simulink model "PubIfDecisionLSM_MDL"  (R2020b)
settings: configuration reference "DspaceConfig" (kept outside this file)
PostLoadFcn:
  | if any(exist('dsrtsu_mdlpostloadfcn', 'file') ~= 0), dsrtsu_mdlpostloadfcn('Execute', bdroot); end
InitFcn:
  | , if any(exist('rtifpga_mdlclblib', 'file') ~= 0), rtifpga_mdlclblib('Init', bdroot); end,
  | , if any(exist('dsmpb_private', 'file') ~= 0), dsmpb_private('dsmpb_mdlclblib', 'Init', bdroot); end,
values from neighbouring files (symbols this model uses):
  P_LSM_ALC_Enable = 0.0    [LSM_Parameter.sldd]
  P_LSM_AwayEdge_offset = 0.1    [LSM_Parameter.sldd]
  P_LSM_CentValidErr = 1.0    [LSM_Parameter.sldd]
  P_LSM_DOP_C0_EN_Limit = 0.8    [LSM_Parameter.sldd]
  P_LSM_DOP_C0_out_Limit = 2.0    [LSM_Parameter.sldd]
  P_LSM_DOP_C1_EN_Limit : value not decoded    [LSM_Parameter.sldd]
  P_LSM_DOP_C1_out_Limit : value not decoded    [LSM_Parameter.sldd]
  P_LSM_DOP_C1AndC2_Lim_X : value not decoded    [LSM_Parameter.sldd]
  P_LSM_DOP_C2_EN_Limit : value not decoded    [LSM_Parameter.sldd]
  P_LSM_DOP_C2_out_Limit : value not decoded    [LSM_Parameter.sldd]
  P_LSM_DOP_In_Pre2Dop_Dis = 1.0    [LSM_Parameter.sldd]
  P_LSM_DOP_Out_Pre2Dop_Dis = 2.0    [LSM_Parameter.sldd]
  P_LSM_DOP_PreDis_X : value not decoded    [LSM_Parameter.sldd]
  P_LSM_DOP_PreDis_Y : value not decoded    [LSM_Parameter.sldd]
  P_LSM_DOPEnableSW = 1.0    [LSM_Parameter.sldd]
  P_LSM_DOPValid_CheckTime = 0.06    [LSM_Parameter.sldd]
  P_LSM_DoubleLine_Curr2Cent_Dislimit = 0.5    [LSM_Parameter.sldd]
  P_LSM_DoubleLine_Dop2Cent_Dislimit = 0.5    [LSM_Parameter.sldd]
  P_LSM_DoubleLine_DOPOut_C1 : value not decoded    [LSM_Parameter.sldd]
  P_LSM_DoubleLine_Pre2Cent_Dislimit = 1.0    [LSM_Parameter.sldd]
  P_LSM_Error_Limit = 0.5    [LSM_Parameter.sldd]
  P_LSM_IFV2CenterAxis = 0.0    [LSM_Parameter.sldd]
  P_LSM_IFV2RearAxis = 0.0    [LSM_Parameter.sldd]
  P_LSM_Line2Edge_limit = 0.5    [LSM_Parameter.sldd]
  P_LSM_Line_Error = 0.1    [LSM_Parameter.sldd]
  P_LSM_LineSTD_Limit = 0.15    [LSM_Parameter.sldd]
  P_LSM_NOH_Switch = 0.0    [LSM_Parameter.sldd]
  P_LSM_OTL_C0_Factor = 1.0    [LSM_Parameter.sldd]
  P_LSM_OTL_C1_Factor = 0.5    [LSM_Parameter.sldd]
  P_LSM_OTL_C2_Factor = 0.5    [LSM_Parameter.sldd]
  P_LSM_Pre2OnlyLineDis = 5.0    [LSM_Parameter.sldd]
  P_LSM_Pre_t = 0.0    [LSM_Parameter.sldd]
  P_LSM_SingleLine_Cent2Edge_Dislimit = 100.0    [LSM_Parameter.sldd]
  P_LSM_SingleLine_Curr2Cent_Dislimit = 0.2    [LSM_Parameter.sldd]
  P_LSM_SingleLine_Dop2Cent_Dislimit = 0.2    [LSM_Parameter.sldd]
  P_LSM_SingleLine_DOPOut_C1 : value not decoded    [LSM_Parameter.sldd]
  P_LSM_SingleLine_Pre2Cent_Dislimit = 0.5    [LSM_Parameter.sldd]
  P_LSM_TJALimitSpd = 60.0    [LSM_Parameter.sldd]
undefined symbols (not defined in the file or in its folder): P_lCS_IFV2CenterAxis, P_LCS_IFV2RearAxis, P_LSM_EntryEdge_offset, P_LSM_EntryLnChngEnSwitch, P_LSM_EntryVanishDis, P_LSM_LinetLostTime, P_LSM_LineWijCal_C12, P_LSM_LineWijCal_C13, P_LSM_MapValid_ErrorSwitch, P_LSM_PosLineLcFac, P_LSM_SpdLim_Stub_Spd, P_LSM_SpdLim_StubLength, P_LSM_SpdTurnAlarm
libraries: simulink x324, TrueDurationTime x11
(part 9 of 25)

== system PubIfDecisionLSM_MDL/Subsystem1/TargetLineCalc_20ms/TargetLineCalc/Subsystem5 ==
  kap : Inport
  vRef : Inport  Port=2
  preDis : Inport  Port=3
  RoadWidth1 : Inport  Port=4
  <CentLineValid> : Inport  Port=5
  <CentLineC3> : Inport  Port=6
  <CentLineC2> : Inport  Port=7
  <CentLineC1> : Inport  Port=8
  <CentLineC0> : Inport  Port=9
  Conf : Inport  Port=10
  <A3> : Inport  Port=11
  <A2> : Inport  Port=12
  <A1> : Inport  Port=13
  <A0> : Inport  Port=14
  <LineReliable> : Inport  Port=15
  <Range> : Inport  Port=16
  CosOfPsi : Inport  Port=17
  SinOfPsi : Inport  Port=18
  dDeltaX : Inport  Port=19
  dDeltaY : Inport  Port=20
  HWASts : Inport  Port=21
  1-D Lookup Table3 : Lookup_n-D  NumberOfTableDimensions=1  BreakpointsForDimension1=[0 0.0001 0.0005 0.001 0.005 0.01 0.05]  Table=[0 0.1 0.3 0.6 0.8 0.8 0.8]  InternalRulePriority=Speed  RndMeth=Simplest  InputSameDT=on
  1-D Lookup Table4 : Lookup_n-D  NumberOfTableDimensions=1  BreakpointsForDimension1=[0 0.0001 0.0005 0.001 0.005 0.01 0.05]  Table=[0 0.1 0.3 0.6 0.8 0.8 0.8]  InternalRulePriority=Speed  RndMeth=Simplest  InputSameDT=on
  1-D Lookup Table5 : Lookup_n-D  NumberOfTableDimensions=1  BreakpointsForDimension1=[0 0.1 0.3 0.5 0.7 0.9 1]  Table=[0 0.1 0.2 0.4 0.7 1 1]  InternalRulePriority=Speed  RndMeth=Simplest  InputSameDT=on
  1-D Lookup Table6 : Lookup_n-D  NumberOfTableDimensions=1  BreakpointsForDimension1=[0 0.1 0.3 0.5 0.7 0.9 1]  Table=[0 0.1 0.2 0.4 0.7 1 1]  InternalRulePriority=Speed  RndMeth=Simplest  InputSameDT=on
  2-D Lookup Table : Lookup_n-D  BreakpointsForDimension1=[20,50,100,120]  BreakpointsForDimension2=[0,0.2,0.4,0.6,0.8,1,1.2,1.4,1.6,1.8,2,2.5,3]  Table=reshape([1,1,1,1,1,1,1,1,1,1,1,1,1,1,1,0.8,1,0.9,0.5,0.4,1,0.8,0.3,0.2,1,0.7,0.1,0.1,1,0.6,0,0,0.8,0.5,0,0,0.7,0.3,0,0,0.6,0,0,0,0.3,0,0,0,0,0,0,0],4,13)  InternalRulePriority=Speed  RndMeth=Simplest  InputSameDT=on
      settings: InputPortMap=u0,u1
  2-D Lookup Table1 : Lookup_n-D  BreakpointsForDimension1=[20,50,100,120]  BreakpointsForDimension2=[0,0.2,0.4,0.6,0.8,1,1.2,1.4,1.6,1.8,2,2.5,3]  Table=reshape([1,1,1,1,1,1,1,1,1,1,1,1,1,1,1,0.8,1,0.9,0.5,0.4,1,0.8,0.3,0.2,1,0.7,0.1,0.1,1,0.6,0,0,0.8,0.5,0,0,0.7,0.3,0,0,0.6,0,0,0,0.3,0,0,0,0,0,0,0],4,13)  InternalRulePriority=Speed  RndMeth=Simplest  InputSameDT=on
      settings: InputPortMap=u0,u1
  2-D Lookup Table2 : Lookup_n-D  Commented=on  BreakpointsForDimension1=[20,50,100]  BreakpointsForDimension2=[0,0.2,0.4,0.6,0.8,1,1.2,1.4,1.6,1.8,2,2.5,3]  Table=reshape([1,1,1,1,1,1,1,1,0.9,1,1,0.5,1,0.9,0.3,1,0.8,0.2,1,0.7,0.1,1,0.6,0,0.8,0.5,0,0.7,0.3,0,0.6,0.1,0,0.3,0,0,0,0,0],3,13)  InternalRulePriority=Speed  RndMeth=Simplest  InputSameDT=on
      settings: InputPortMap=u0,u1
  2-D Lookup Table3 : Lookup_n-D  BreakpointsForDimension1=[10,50,80,120]  BreakpointsForDimension2=[0,5,10,20,40,50,60,80,100]  Table=reshape([0,0,0,0,0,0,0,0,0.4,0.2,0,0,0.6,0.4,0.2,0,1,0.6,0.5,0.3,1,0.8,0.7,0.5,1,1,0.9,0.8,1,1,1,1,1,1,1,1],4,9)  InternalRulePriority=Speed  RndMeth=Simplest  InputSameDT=on
      settings: InputPortMap=u0,u1
  2-D Lookup Table4 : Lookup_n-D  BreakpointsForDimension1=[10,50,80,120]  BreakpointsForDimension2=[0,5,10,20,40,50,60,80,100]  Table=reshape([0,0,0,0,0,0,0,0,0.4,0.2,0,0,0.6,0.4,0.2,0,1,0.6,0.5,0.3,1,0.8,0.7,0.5,1,1,0.9,0.8,1,1,1,1,1,1,1,1],4,9)  InternalRulePriority=Speed  RndMeth=Simplest  InputSameDT=on
      settings: InputPortMap=u0,u1
  <A2>1 : InportShadow  Port=12
  Abs2 : Abs
  Abs3 : Abs
  Add : Sum  Inputs=+++
  Add1 : Sum  Inputs=+++
  Constant10 : Constant  Value=[0,0,0.2,0.5,0.8,1,1,1,1,0.3,0,0]
  Constant11 : Constant  Value=[-1.2,-0.2,0,0.5,1,1.3,1.5,2.1,2.3,3.5,4,5]
  Constant12 : Constant  Value=3.75
  Constant13 : Constant  Value=[0,0,0.2,0.5,0.8,1,1,1,1,0.3,0,0]
  Constant14 : Constant  Value=[-1.2,-0.2,0,0.5,1,1.3,1.5,2.1,2.3,3.5,4,5]
  Constant15 : Constant  Value=3.75
  Constant16 : Constant  Value=1.3  OutDataTypeStr=single
  Constant21 : Constant  Value=1.3  OutDataTypeStr=single
  Constant7 : Constant  Value=P_LSM_LineWijCal_C12
  Constant9 : Constant  Value=P_LSM_LineWijCal_C13
  Gain1 : Gain  Gain=3.6
  Gain2 : Gain  Gain=1.03
  Gain3 : Gain  Gain=3.6
  Gain4 : Gain  Gain=1.03
  If : If
  If Action Subsystem : Subsystem  TreatAsAtomicUnit=on
  If Action Subsystem1 : Subsystem  TreatAsAtomicUnit=on
  If Action Subsystem2 : Subsystem  TreatAsAtomicUnit=on
  If Action Subsystem3 : Subsystem  TreatAsAtomicUnit=on
  If Action Subsystem4 : Subsystem  TreatAsAtomicUnit=on
  If Action Subsystem5 : Subsystem  TreatAsAtomicUnit=on
  If1 : If
  If2 : If
  Lookup Table Dynamic : simulink/Lookup Tables/Lookup Table Dynamic  LookUpMeth=Interpolation-Use End Values  OutDataType=fixdt('single')  OutScaling=[]  OutputDataTypeScalingMode=Specify via dialog  OutDataTypeStr=single  DoSatur=off
  Lookup Table Dynamic1 : simulink/Lookup Tables/Lookup Table Dynamic  LookUpMeth=Interpolation-Use End Values  OutDataType=fixdt('single')  OutScaling=[]  OutputDataTypeScalingMode=Specify via dialog  OutDataTypeStr=single  DoSatur=off
  MATLAB Function2 : MATLAB Function  TreatAsAtomicUnit=on
  MATLAB Function3 : MATLAB Function  TreatAsAtomicUnit=on
  MATLAB Function6 : MATLAB Function  TreatAsAtomicUnit=on
  MATLAB Function7 : MATLAB Function  TreatAsAtomicUnit=on
  MATLAB Function8 : MATLAB Function  TreatAsAtomicUnit=on
  Merge{,1..3} (4 alike) : Merge
  Product{,1..7} (8 alike) : Product
  Product8 : Product  Inputs=**/
  Product9 : Product  Inputs=**/
  RoadWidth1_1 : InportShadow  Port=4
  Saturation : Saturate  UpperLimit=single(5)  LowerLimit=single(2.4)
  Saturation1 : Saturate  UpperLimit=single(5)  LowerLimit=single(2.4)
  Selector2 : Selector  InputPortWidth=4  IndexOptions=Index vector (dialog)  Indices=2  OutputSizes=1
  Selector3 : Selector  InputPortWidth=4  IndexOptions=Index vector (dialog)  Indices=3  OutputSizes=1
  Selector4 : Selector  InputPortWidth=4  IndexOptions=Index vector (dialog)  Indices=2  OutputSizes=1
  Selector5 : Selector  InputPortWidth=4  IndexOptions=Index vector (dialog)  Indices=3  OutputSizes=1
  Selector6 : Selector  InputPortWidth=4  IndexOptions=Index vector (dialog)  Indices=2  OutputSizes=1
  Selector7 : Selector  InputPortWidth=4  IndexOptions=Index vector (dialog)  Indices=3  OutputSizes=1
  Sum : Sum  Inputs=|++
  Sum1 : Sum  Inputs=|++
  Unit Delay : UnitDelay  SampleTime=-1  HasFrameUpgradeWarning=on
  Unit Delay1 : UnitDelay  SampleTime=-1  HasFrameUpgradeWarning=on
  vRef_1 : InportShadow  Port=2
  LH1Wij : Outport
  LH2Wij : Outport  Port=2
  wires:
  Saturation1/1 -> Product9/2
  RoadWidth1/1 -> Saturation/1
  [LH22] -> Product2/1
  Lookup Table Dynamic1/1 -> Product4/1
  Gain1/1 -> Gain2/1
  [LH21] -> Product1/1
  <CentLineC0>/1 -> MATLAB Function6/7(CentLineC0K1)
  Gain2/1 -> Sum1/1
  Product/1 -> [LH21]
  <Range>/1 -> Selector3/1, Selector2/1
  Saturation/1 -> Product8/2
  vRef_1/1 -> Gain1/1
  MATLAB Function6/1(d_cur2) -> Lookup Table Dynamic/1
  2-D Lookup Table1/1 -> Product4/2
  <LineReliable>/1 -> MATLAB Function8/1(VisLineReliable)
  Sum1/1 -> 2-D Lookup Table4/1, 2-D Lookup Table3/1
  Product5/1 -> Add1/1
  1-D Lookup Table5/1 -> [LH23]
  Product7/1 -> Add1/3
  [LH33] -> Product7/1
  dDeltaX/1 -> MATLAB Function6/16(dDeltaX)
  MATLAB Function8/2(dy3_Rel) -> 1-D Lookup Table6/1
  Constant16/1 -> Sum/2
  Constant13/1 -> Lookup Table Dynamic1/3
  Constant21/1 -> Sum1/2
  MATLAB Function3/1(Fac1) -> [Fac1]
  2-D Lookup Table3/1 -> [LH22]
  Sum/1 -> 2-D Lookup Table1/1, 2-D Lookup Table/1
  Constant12/1 -> Product8/3
  [Fac3] -> Product7/2
  [Fac1] -> Product5/2
  [Fac2] -> Product6/2
  <CentLineC2>/1 -> MATLAB Function6/5(CentLineC2K1)
  [LH23] -> Product3/1
  SinOfPsi/1 -> MATLAB Function6/15(SinOfPsi)
  Product8/1 -> Lookup Table Dynamic/2
  1-D Lookup Table6/1 -> [LH33]
  Product2/1 -> Add/2
  [Fac1] -> Product1/2
  Product1/1 -> Add/1
  2-D Lookup Table/1 -> Product/2
  <CentLineC1>/1 -> MATLAB Function6/6(CentLineC1K1)
  Selector2/1 -> MATLAB Function7/1(L2_R)
  Product9/1 -> Lookup Table Dynamic1/2
  Gain3/1 -> Gain4/1
  <A0>/1 -> MATLAB Function6/11(VisLineA0)
  Constant11/1 -> Product8/1
  Product6/1 -> Add1/2
  Gain4/1 -> Sum/1
  MATLAB Function6/3(d_cur3) -> Lookup Table Dynamic1/1
  MATLAB Function6/2(delta_d2) -> 2-D Lookup Table/2
  RoadWidth1_1/1 -> Saturation1/1
  Constant14/1 -> Product9/1
  Lookup Table Dynamic/1 -> Product/1
  Constant10/1 -> Lookup Table Dynamic/3
  <CentLineC3>/1 -> MATLAB Function6/4(CentLineC3K1)
  [LH32] -> Product6/1
  MATLAB Function6/4(delta_d3) -> 2-D Lookup Table1/2
  [Fac2] -> Product2/2
  Constant9/1 -> MATLAB Function3/2(C13)
  [LH31] -> Product5/1
  [Fac3] -> Product3/2
  Constant7/1 -> MATLAB Function3/1(C12)
  Constant15/1 -> Product9/3
  MATLAB Function7/1(dy2_Ran) -> 2-D Lookup Table3/2
  MATLAB Function8/1(dy2_Rel) -> 1-D Lookup Table5/1
  preDis/1 -> MATLAB Function6/2(preDis)
  MATLAB Function3/2(Fac2) -> [Fac2]
  Product4/1 -> [LH31]
  vRef/1 -> Gain3/1
  MATLAB Function3/3(Fac3) -> [Fac3]
  kap/1 -> MATLAB Function6/1(kap)
  2-D Lookup Table4/1 -> [LH32]
  MATLAB Function7/2(dy3_Ran) -> 2-D Lookup Table4/2
  Product3/1 -> Add/3
  <A2>/1 -> MATLAB Function6/9(VisLineA2)
  Selector3/1 -> MATLAB Function7/2(L3_R)
  CosOfPsi/1 -> MATLAB Function6/14(CosOfPsi)
  <A1>/1 -> MATLAB Function6/10(VisLineA1)
  <A3>/1 -> MATLAB Function6/8(VisLineA3)
  dDeltaY/1 -> MATLAB Function6/17(dDeltaY)
  Conf/1 -> Selector5/1, Selector4/1
  Selector5/1 -> If1/1
  Selector4/1 -> If/1
  Add/1 -> If Action Subsystem/1(In1)
  If/2 -> If Action Subsystem2/Action
  Merge/1 -> LH1Wij/1
  If Action Subsystem/1(LH1Wij) -> Merge/1
  If Action Subsystem2/1(LH1Wij) -> Merge/2
  If Action Subsystem3/1(LH1Wij) -> Merge1/2
  If Action Subsystem1/1(LH1Wij) -> Merge1/1
  Merge1/1 -> LH2Wij/1
  Add1/1 -> If Action Subsystem1/1(In1)
  If1/2 -> If Action Subsystem3/Action
  If/1 -> If Action Subsystem/Action
  If1/1 -> If Action Subsystem1/Action
  <CentLineValid>/1 -> MATLAB Function6/3(CentLineValidK1)
  If Action Subsystem5/2(Out2) -> Merge3/1
  1-D Lookup Table4/1 -> If Action Subsystem4/1(In1)
  If2/2 -> If Action Subsystem4/Action
  If Action Subsystem4/2(Out2) -> Merge3/2
  Merge2/1 -> MATLAB Function6/12(n1)
  If Action Subsystem4/1(Out1) -> Merge2/2
  Abs2/1 -> 1-D Lookup Table4/1
  <A2>1/1 -> Selector7/1, Selector6/1
  Abs3/1 -> 1-D Lookup Table3/1
  1-D Lookup Table3/1 -> If Action Subsystem4/2(In2)
  If2/1 -> If Action Subsystem5/Action
  If Action Subsystem5/1(Out1) -> Merge2/1
  Merge3/1 -> MATLAB Function6/13(n2)
  Selector6/1 -> Abs2/1
  Selector7/1 -> Abs3/1
  Unit Delay1/1 -> MATLAB Function2/2(HWAStsK1)
  HWASts/1 -> MATLAB Function6/18(HWASts), MATLAB Function2/1(HWASts), Unit Delay1/1
  MATLAB Function2/1(Changelane) -> If2/1
  MATLAB Function2/2(Lock_counter) -> Unit Delay/1
  Unit Delay/1 -> MATLAB Function2/3(Lock_counterK1)

== system PubIfDecisionLSM_MDL/Subsystem1/TargetLineCalc_20ms/TargetLineCalc/TypeConf ==
  LeftType : Inport
  LeftDLMType : Inport  Port=2
  LeftDECELType : Inport  Port=3
  RightType : Inport  Port=4
  RightDLMType : Inport  Port=5
  RightDECELType : Inport  Port=6
  Line_update : Inport  Port=7
  LeftColor : Inport  Port=8
  LLeftType : Inport  Port=9
  MATLAB Function : MATLAB Function  TreatAsAtomicUnit=on
  RoadWidthCalc1 : MATLAB Function  TreatAsAtomicUnit=on
  Unit Delay{,1..7,36..37} (10 alike) : UnitDelay  SampleTime=-1  HasFrameUpgradeWarning=on
  Out1 : Outport
  Out2 : Outport  Port=2
  wires:
  MATLAB Function/7(LeftColor) -> Unit Delay6/1
  MATLAB Function/4(RightType) -> RoadWidthCalc1/4(RightType), Unit Delay2/1
  LeftColor/1 -> MATLAB Function/8(LeftColor_en)
  Unit Delay3/1 -> MATLAB Function/14(RightDLMTypeK1)
  Unit Delay7/1 -> MATLAB Function/17(LLeftType_enK1)
  Unit Delay6/1 -> MATLAB Function/16(LeftColor_enK1)
  LeftDLMType/1 -> MATLAB Function/3(LeftDLMType_en)
  Unit Delay5/1 -> MATLAB Function/12(LeftDECELTypeK1)
  Unit Delay4/1 -> MATLAB Function/15(RightDECELTypeK1)
  Unit Delay2/1 -> MATLAB Function/13(RightTypeK1)
  MATLAB Function/8(LLeftType) -> Unit Delay7/1
  Unit Delay1/1 -> MATLAB Function/11(LeftDLMTypeK1)
  LeftDECELType/1 -> MATLAB Function/4(LeftDECELType_en)
  RightDECELType/1 -> MATLAB Function/7(RightDECELType_en)
  MATLAB Function/6(RightDECELType) -> RoadWidthCalc1/6(RightDECELType), Unit Delay4/1
  MATLAB Function/5(RightDLMType) -> RoadWidthCalc1/5(RightDLMType), Unit Delay3/1
  MATLAB Function/1(LeftType) -> Unit Delay/1, RoadWidthCalc1/1(LeftType)
  LLeftType/1 -> MATLAB Function/9(LLeftType_en)
  RoadWidthCalc1/1(LeftEn) -> Out1/1
  Unit Delay36/1 -> RoadWidthCalc1/8(Cnt2K1)
  Unit Delay37/1 -> RoadWidthCalc1/7(Cnt1K1)
  MATLAB Function/2(LeftDLMType) -> Unit Delay1/1, RoadWidthCalc1/2(LeftDLMType)
  MATLAB Function/3(LeftDECELType) -> Unit Delay5/1, RoadWidthCalc1/3(LeftDECELType)
  RoadWidthCalc1/4(Cnt2) -> Unit Delay36/1
  RightType/1 -> MATLAB Function/5(RightType_en)
  RoadWidthCalc1/3(Cnt1) -> Unit Delay37/1
  LeftType/1 -> MATLAB Function/2(LeftType_en)
  Unit Delay/1 -> MATLAB Function/10(LeftTypeK1)
  RightDLMType/1 -> MATLAB Function/6(RightDLMType_en)
  Line_update/1 -> MATLAB Function/1(update)
  RoadWidthCalc1/2(RightEn) -> Out2/1

== system PubIfDecisionLSM_MDL/Subsystem1/TargetLineCalc_20ms/TargetLineCalc/TypeConf1 ==
  LeftType : Inport
  RightType : Inport  Port=2
  RoadWidthCalc1 : MATLAB Function  TreatAsAtomicUnit=on
  Unit Delay36 : UnitDelay  SampleTime=-1  HasFrameUpgradeWarning=on
  Unit Delay37 : UnitDelay  SampleTime=-1  HasFrameUpgradeWarning=on
  LeftEn : Outport
  RightEn : Outport  Port=2
  wires:
  RightType/1 -> RoadWidthCalc1/2(RightType)
  Unit Delay36/1 -> RoadWidthCalc1/4(Cnt2K1)
  RoadWidthCalc1/2(RightEn) -> RightEn/1
  LeftType/1 -> RoadWidthCalc1/1(LeftType)
  RoadWidthCalc1/4(Cnt2) -> Unit Delay36/1
  RoadWidthCalc1/3(Cnt1) -> Unit Delay37/1
  Unit Delay37/1 -> RoadWidthCalc1/3(Cnt1K1)
  RoadWidthCalc1/1(LeftEn) -> LeftEn/1

== system PubIfDecisionLSM_MDL/Subsystem1/TargetLineCalc_20ms2/TargetLineCalc/CenLineCal1 ==
  LCKSts : Inport
  kap : Inport  Port=2
  preDis : Inport  Port=3
  VisLine : Inport  Port=4
  VisEdge : Inport  Port=5
  RoadWidth : Inport  Port=6
  LeftLane_change : Inport  Port=7
  RightLane_change : Inport  Port=8
  Bus Creator2 : BusCreator  Inputs=7
  Bus Selector1 : BusSelector  OutputSignals=EdgeConf,EdgeA3,EdgeA2,EdgeA1,EdgeA0
  Bus Selector5 : BusSelector  OutputSignals=LineConf,LineReliable,A3,A2,A1,A0,Range
  Constant : Constant  Value=P_LSM_Line_Error
  Constant1 : Constant  Value=P_LSM_Line2Edge_limit
  Constant2 : Constant  Value=P_LSM_AwayEdge_offset
  Constant3 : Constant  Value=P_LSM_Pre2OnlyLineDis
  Constant4 : Constant  Value=P_LSM_CentValidErr
  Constant5 : Constant  Value=0  OutDataTypeStr=boolean
  Constant6 : Constant  Value=0  OutDataTypeStr=uint8
  Switch : Switch  Criteria=u2 > Threshold
  Switch1 : Switch  Criteria=u2 > Threshold
  Terminator : Terminator
  Unit Delay : UnitDelay  SampleTime=-1  HasFrameUpgradeWarning=on
  Unit Delay1 : UnitDelay  SampleTime=-1  HasFrameUpgradeWarning=on
  centerLineFilter : MATLAB Function  TreatAsAtomicUnit=on
  CenLine : Outport
  Double_Line_Lost : Outport  Port=2
  Line_State : Outport  Port=3
  wires:
  Switch1/1 -> Line_State/1
  Constant6/1 -> Switch1/3
  Switch/1 -> Bus Creator2/1  "CentLineConf"
  Constant5/1 -> Switch/3
  Constant4/1 -> Switch/2, Switch1/2
  Constant3/1 -> centerLineFilter/22(Pre2OnlyLineDis)
  RightLane_change/1 -> centerLineFilter/2(RightLane_change)
  LeftLane_change/1 -> centerLineFilter/1(LeftLane_change)
  centerLineFilter/7(CenLineReliable) -> Bus Creator2/7
  Bus Selector5/2 -> centerLineFilter/10(LineReliable)  "<LineReliable>"
  Constant2/1 -> centerLineFilter/5(Away_offset)
  Constant1/1 -> centerLineFilter/4(Edge_error)
  centerLineFilter/10(Offset) -> Terminator/1  "LSM_Edge_Offset"
  Unit Delay1/1 -> centerLineFilter/24(R_CounterK1)
  Unit Delay/1 -> centerLineFilter/23(L_CounterK1)
  centerLineFilter/12(R_Counter) -> Unit Delay1/1
  centerLineFilter/11(L_Counter) -> Unit Delay/1
  Constant/1 -> centerLineFilter/3(Line_error)
  centerLineFilter/9(Double_Line_Lost) -> Double_Line_Lost/1
  LCKSts/1 -> centerLineFilter/6(LCKSts)
  kap/1 -> centerLineFilter/7(kap)
  RoadWidth/1 -> centerLineFilter/21(RoadWidth)
  Bus Selector1/5 -> centerLineFilter/20(VisEdgeA0)  "<EdgeA0>"
  Bus Selector1/4 -> centerLineFilter/19(VisEdgeA1)  "<EdgeA1>"
  Bus Selector1/3 -> centerLineFilter/18(VisEdgeA2)  "<EdgeA2>"
  Bus Selector1/2 -> centerLineFilter/17(VisEdgeA3)  "<EdgeA3>"
  Bus Selector1/1 -> centerLineFilter/16(VisEdgeConf)  "<EdgeConf>"
  Bus Selector5/7 -> centerLineFilter/15(VisLineR)  "<Range>"
  Bus Selector5/6 -> centerLineFilter/14(VisLineA0)  "<A0>"
  Bus Selector5/1 -> centerLineFilter/9(VisLineConf)  "<LineConf>"
  Bus Selector5/5 -> centerLineFilter/13(VisLineA1)  "<A1>"
  Bus Selector5/3 -> centerLineFilter/11(VisLineA3)  "<A3>"
  Bus Selector5/4 -> centerLineFilter/12(VisLineA2)  "<A2>"
  preDis/1 -> centerLineFilter/8(preDis)
  centerLineFilter/8(Line_State) -> Switch1/1  "LSM_Line_state"
  VisEdge/1 -> Bus Selector1/1
  Bus Creator2/1 -> CenLine/1
  centerLineFilter/5(CentLineC0) -> Bus Creator2/5
  centerLineFilter/3(CentLineC2) -> Bus Creator2/3
  centerLineFilter/1(CentLineConf) -> Switch/1
  centerLineFilter/6(CentLineRange) -> Bus Creator2/6
  VisLine/1 -> Bus Selector5/1
  centerLineFilter/2(CentLineC3) -> Bus Creator2/2
  centerLineFilter/4(CentLineC1) -> Bus Creator2/4

== system PubIfDecisionLSM_MDL/Subsystem1/TargetLineCalc_20ms2/TargetLineCalc/DetectChange ==
  OTLCount : Inport
  Relational Operator : RelationalOperator  Operator=~=  OutDataTypeStr=boolean  RndMeth=Simplest
  Unit Delay49 : UnitDelay  InitialCondition=uint8(0)  SampleTime=-1  HasFrameUpgradeWarning=on
  Out1 : Outport
  wires:
  Relational Operator/1 -> Out1/1
  OTLCount/1 -> Unit Delay49/1, Relational Operator/2
  Unit Delay49/1 -> Relational Operator/1

== system PubIfDecisionLSM_MDL/Subsystem1/TargetLineCalc_20ms2/TargetLineCalc/DetectChange1 ==
  In1 : Inport
  Constant : Constant  Value=0  OutDataTypeStr=uint8
  Relational Operator1 : RelationalOperator  Operator=~=  OutDataTypeStr=boolean  RndMeth=Simplest
  Switch : Switch  Criteria=u2 > Threshold
  Unit Delay68 : UnitDelay  SampleTime=-1  HasFrameUpgradeWarning=on
  Out1 : Outport
  wires:
  Constant/1 -> Switch/3
  Switch/1 -> Out1/1
  Relational Operator1/1 -> Switch/2
  In1/1 -> Relational Operator1/1, Switch/1, Unit Delay68/1
  Unit Delay68/1 -> Relational Operator1/2

== system PubIfDecisionLSM_MDL/Subsystem1/TargetLineCalc_20ms2/TargetLineCalc/DetectIncrease ==
  In : Inport
  Relational Operator : RelationalOperator  Operator=>  OutDataTypeStr=boolean  RndMeth=Simplest
  Unit Delay67 : UnitDelay  SampleTime=-1  HasFrameUpgradeWarning=on
  Out : Outport
  wires:
  Relational Operator/1 -> Out/1
  In/1 -> Relational Operator/1, Unit Delay67/1
  Unit Delay67/1 -> Relational Operator/2

== system PubIfDecisionLSM_MDL/Subsystem1/TargetLineCalc_20ms2/TargetLineCalc/DetectIncrease1 ==
  In : Inport
  Relational Operator : RelationalOperator  Operator=>  OutDataTypeStr=boolean  RndMeth=Simplest
  Unit Delay67 : UnitDelay  SampleTime=-1  HasFrameUpgradeWarning=on
  out : Outport
  wires:
  Unit Delay67/1 -> Relational Operator/2
  In/1 -> Unit Delay67/1, Relational Operator/1
  Relational Operator/1 -> out/1

== system PubIfDecisionLSM_MDL/Subsystem1/TargetLineCalc_20ms2/TargetLineCalc/Subsystem ==
  Spd : Inport
  Compare To Constant22 : simulink/Logic and Bit Operations/Compare To Constant  relop=<  const=1  OutDataTypeStr=boolean
  Constant21 : Constant  Value=0xff
  Switch10 : Switch
  Out1 : Outport
  wires:
  Switch10/1 -> Out1/1
  Constant21/1 -> Switch10/1
  Spd/1 -> Switch10/3, Compare To Constant22/1
  Compare To Constant22/1 -> Switch10/2

== system PubIfDecisionLSM_MDL/Subsystem1/TargetLineCalc_20ms2/TargetLineCalc/Subsystem1 ==
  Dis : Inport
  Compare To Constant1 : simulink/Logic and Bit Operations/Compare To Constant  relop=>  const=2000  OutDataTypeStr=boolean
  Compare To Constant22 : simulink/Logic and Bit Operations/Compare To Constant  relop=<  const=1  OutDataTypeStr=boolean
  Constant21 : Constant  Value=0xffff
  OR : Logic  Operator=OR  AllPortsSameDT=off  OutDataTypeStr=boolean
  Switch10 : Switch
  Out1 : Outport
  wires:
  OR/1 -> Switch10/2
  Compare To Constant1/1 -> OR/2
  Compare To Constant22/1 -> OR/1
  Dis/1 -> Compare To Constant22/1, Compare To Constant1/1, Switch10/3
  Constant21/1 -> Switch10/1
  Switch10/1 -> Out1/1

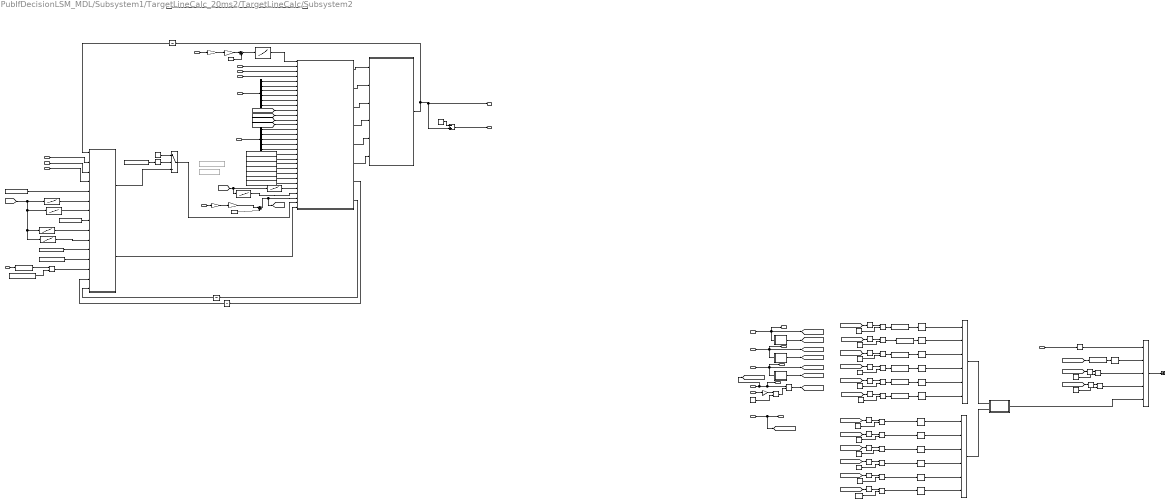
== system PubIfDecisionLSM_MDL/Subsystem1/TargetLineCalc_20ms2/TargetLineCalc/Subsystem2 ==
  LCKSts : Inport
  Line_State : Inport  Port=2
  vRef : Inport  Port=3
  DOP_Valid : Inport  Port=4
  DOP_C3 : Inport  Port=5
  DOP_C2 : Inport  Port=6
  DOP_C1 : Inport  Port=7
  DOP_C0 : Inport  Port=8
  DOP_Range : Inport  Port=9
  CentLine : Inport  Port=10
  EdgeLine : Inport  Port=11
  kap : Inport  Port=12
  Abs{,1,3..14} (14 alike) : Abs
  Bus Selector1 : BusSelector  OutputSignals=EdgeConf,EdgeA3,EdgeA2,EdgeA1,EdgeA0
  Bus Selector6 : BusSelector  OutputSignals=CentLineConf,CentLineC3,CentLineC2,CentLineC1,CentLineC0,CentLineRange
  C0max : Constant  Value=1.5  OutDataTypeStr=single
  C0th : Constant  Value=0.9  OutDataTypeStr=single
  C0th1 : Constant  Value=0.6  OutDataTypeStr=single
  C1max:30° : Constant  Value=0.58  OutDataTypeStr=single
  C1th:10° : Constant  Value=0.176  OutDataTypeStr=single
  C1th:10°1 : Constant  Value=0.08  OutDataTypeStr=single
  C2th : Constant  Value=0.008  OutDataTypeStr=single
  C2th1 : Constant  Value=0.006  OutDataTypeStr=single
  Chart : Stateflow chart  TreatAsAtomicUnit=on
      settings: PortSchema="{\"entries\":[{\"content\":{\"sides\":[{\"content\":{\"connectorIds\":[\"In2\",\"In1\"]},\"type\":\"ConnectorPlacement.EquallySpacedRectSide\",\"uuid\":\"e53ab263-18d4-4398-8fad-2a536e7c737c\"},{\"content\":{\"connectorIds\":[\"Out1\"],\"side\":\"RIGHT\"},\"type\":\"ConnectorPlacement.EquallySpacedRectSide\",\"uuid\":\"b2acecce-e73e-419a-a9e7-11eb92620f5a\"},{\"content\":{\"connectorIds\":[],\"side\":\"TOP\"},\"type\":\"ConnectorPlacement.EquallySpacedRectSide\",\"uuid\":\"8139e609-291b-42df-ade2-518731258890\"},{\"content\":{\"connectorIds\":[],\"side\":\"HIDDEN\"},\"type\":\"ConnectorPlacement.EquallySpacedRectSide\",\"uuid\":\"25f8d80a-ba71-4848-a7f0-1c840b95c0bf\"}]},\"type\":\"ConnectorPlacement.EquallySpacedConnector\",\"uuid\":\"d97a9ee1-ef81-44f0-bee3-63dee7baeb52\"}],\"packageUris\":[\"http://schema.mathworks.com/mf0/Connector/R2020b\"],\"version\":\"1.0\"}"
  Compare To Constant{,1,9..14} (8 alike) : simulink/Logic and Bit Operations/Compare To Constant  relop===  const=1  OutDataTypeStr=boolean
  Compare To Constant{2,4,6,8} (4 alike) : simulink/Logic and Bit Operations/Compare To Constant  relop=>  const=0.1  OutDataTypeStr=boolean
  Compare To Constant3 : simulink/Logic and Bit Operations/Compare To Constant  relop=>  const=0.06  OutDataTypeStr=boolean
  Compare To Constant5 : simulink/Logic and Bit Operations/Compare To Constant  relop=>  const=0.06  OutDataTypeStr=boolean
  Compare To Constant7 : simulink/Logic and Bit Operations/Compare To Constant  relop=>  const=0.06  OutDataTypeStr=boolean
  Constant : Constant  Value=P_LSM_DOPEnableSW
  Constant1 : Constant  OutDataTypeStr=boolean
  Constant10 : Constant  Commented=on  Value=P_LSM_Error_Limit
  Constant11 : Constant  Value=1.3  OutDataTypeStr=single
  Constant12 : Constant  Commented=on  Value=P_LSM_TJALimitSpd
  Constant13 : Constant  Value=P_LSM_DoubleLine_Dop2Cent_Dislimit
  Constant14 : Constant  Value=P_LSM_DOP_In_Pre2Dop_Dis
  Constant15 : Constant  OutDataTypeStr=uint8
  Constant16 : Constant  Value=P_LSM_SingleLine_Cent2Edge_Dislimit
  Constant17 : Constant  Value=P_LSM_SingleLine_Pre2Cent_Dislimit
  Constant18 : Constant  Value=P_LSM_SingleLine_Curr2Cent_Dislimit
  Constant19 : Constant  Value=P_LSM_DoubleLine_Pre2Cent_Dislimit
  Constant2 : Constant  Value=25  OutDataTypeStr=single
  Constant20 : Constant  Value=P_LSM_DoubleLine_Curr2Cent_Dislimit
  Constant21 : Constant  Value=P_LSM_SingleLine_Dop2Cent_Dislimit
  Constant22 : Constant  Value=P_LSM_DOP_Out_Pre2Dop_Dis
  Constant23 : Constant  Value=P_LSM_DOPValid_CheckTime
  Constant3 : Constant  Value=P_LSM_DOP_C0_EN_Limit
  Constant6 : Constant  Value=P_LSM_DOP_C0_out_Limit
  Constant9 : Constant  Value=1.3  OutDataTypeStr=single
  DOP_C4 : InportShadow  Port=8
  DOP_C5 : InportShadow  Port=7
  DOP_C6 : InportShadow  Port=6
  DOP_Valid1 : InportShadow  Port=4
  DOP_Valid2 : InportShadow  Port=4
  Gain : Gain  Gain=5  OutDataTypeStr=single
  Gain1 : Gain  Gain=3.6
  Gain2 : Gain  Gain=1.03
  Gain3 : Gain  Gain=3.6
  Gain4 : Gain  Gain=1.03
  LineSelect1 : MATLAB Function  TreatAsAtomicUnit=on
  Logical Operator : Logic  Inputs=5  AllPortsSameDT=off  OutDataTypeStr=boolean
  Logical Operator2 : Logic  Operator=OR  Inputs=6  AllPortsSameDT=off  OutDataTypeStr=boolean
  Logical Operator3 : Logic  Inputs=6  AllPortsSameDT=off  OutDataTypeStr=boolean
  MATLAB Function : MATLAB Function  TreatAsAtomicUnit=on
  Max : MinMax  Function=max  Inputs=2
  Relational Operator{,1..2,10..15} (9 alike) : RelationalOperator  Operator=<=  OutDataTypeStr=boolean  RndMeth=Simplest
  Relational Operator3 : RelationalOperator  Operator=>  OutDataTypeStr=boolean  RndMeth=Simplest
  Relational Operator{4..9} (6 alike) : RelationalOperator  OutDataTypeStr=boolean  RndMeth=Simplest
  Subsystem1 : Subsystem
  Subsystem2 : Subsystem
  Subsystem3 : Subsystem
  Subtract : Sum  Inputs=-+
  Sum : Sum  Inputs=|++
  Sum1 : Sum  Inputs=|++
  Switch : Switch  Criteria=u2 ~= 0
  TJA_Line_Select : Stateflow chart  TreatAsAtomicUnit=on
      settings: PortSchema="{\"entries\":[{\"content\":{\"sides\":[{\"content\":{\"connectorIds\":[\"In4\",\"In5\",\"In1\",\"In3\",\"In6\",\"In2\"]},\"type\":\"ConnectorPlacement.EquallySpacedRectSide\",\"uuid\":\"94136a59-7eb8-456e-b1b6-1f0641166e38\"},{\"content\":{\"connectorIds\":[\"Out1\"],\"side\":\"RIGHT\"},\"type\":\"ConnectorPlacement.EquallySpacedRectSide\",\"uuid\":\"664f3682-a903-47ba-a547-cb8bac6665aa\"},{\"content\":{\"connectorIds\":[],\"side\":\"TOP\"},\"type\":\"ConnectorPlacement.EquallySpacedRectSide\",\"uuid\":\"464c275d-d572-4c7f-987d-e7fbd4ad7b48\"},{\"content\":{\"connectorIds\":[],\"side\":\"HIDDEN\"},\"type\":\"ConnectorPlacement.EquallySpacedRectSide\",\"uuid\":\"4c0a197a-3630-40df-8db9-9313a36d3a51\"}]},\"type\":\"ConnectorPlacement.EquallySpacedConnector\",\"uuid\":\"5cfbbf76-c0d2-41e2-9bfb-a7f0229f0d71\"}],\"packageUris\":[\"http://schema.mathworks.com/mf0/Connector/R2020b\"],\"version\":\"1.0\"}"
  Terminator : Terminator
  TrueDurationTime{1..8} (8 alike) : TrueDurationTime/TrueDurationTime  TCycle=0.02
  Unit Delay : UnitDelay  SampleTime=-1  HasFrameUpgradeWarning=on
  Unit Delay1 : UnitDelay  SampleTime=-1  HasFrameUpgradeWarning=on
  Unit Delay2 : UnitDelay  SampleTime=-1  HasFrameUpgradeWarning=on
  dC0th : Constant  Value=0.6  OutDataTypeStr=single
  dC0th1 : Constant  Value=0.3  OutDataTypeStr=single
  dC1th:2.5°/s : Constant  Value=0.045  OutDataTypeStr=single
  dC1th:2.5°/s1 : Constant  Value=0.02  OutDataTypeStr=single
  dC2th : Constant  Value=0.001  OutDataTypeStr=single
  dC2th1 : Constant  Value=0.0005  OutDataTypeStr=single
  preDisMinTable : Lookup_n-D  NumberOfTableDimensions=1  BreakpointsForDimension1=P_LSM_DOP_PreDis_X  Table=P_LSM_DOP_PreDis_Y  ExtrapMethod=Clip  InternalRulePriority=Speed  RndMeth=Simplest  InputSameDT=on
  preDisMinTable1 : Lookup_n-D  NumberOfTableDimensions=1  BreakpointsForDimension1=P_LSM_DOP_C1AndC2_Lim_X  Table=P_LSM_DOP_C1_EN_Limit  ExtrapMethod=Clip  InternalRulePriority=Speed  RndMeth=Simplest  InputSameDT=on
  preDisMinTable2 : Lookup_n-D  NumberOfTableDimensions=1  BreakpointsForDimension1=P_LSM_DOP_C1AndC2_Lim_X  Table=P_LSM_DOP_C2_EN_Limit  ExtrapMethod=Clip  InternalRulePriority=Speed  RndMeth=Simplest  InputSameDT=on
  preDisMinTable3 : Lookup_n-D  NumberOfTableDimensions=1  BreakpointsForDimension1=P_LSM_DOP_C1AndC2_Lim_X  Table=P_LSM_DOP_C1_out_Limit  ExtrapMethod=Clip  InternalRulePriority=Speed  RndMeth=Simplest  InputSameDT=on
  preDisMinTable4 : Lookup_n-D  NumberOfTableDimensions=1  BreakpointsForDimension1=P_LSM_DOP_C1AndC2_Lim_X  Table=P_LSM_DOP_C2_out_Limit  ExtrapMethod=Clip  InternalRulePriority=Speed  RndMeth=Simplest  InputSameDT=on
  preDisMinTable5 : Lookup_n-D  NumberOfTableDimensions=1  BreakpointsForDimension1=P_LSM_DOP_C1AndC2_Lim_X  Table=P_LSM_DoubleLine_DOPOut_C1  ExtrapMethod=Clip  InternalRulePriority=Speed  RndMeth=Simplest  InputSameDT=on
  preDisMinTable7 : Lookup_n-D  NumberOfTableDimensions=1  BreakpointsForDimension1=P_LSM_DOP_C1AndC2_Lim_X  Table=P_LSM_SingleLine_DOPOut_C1  ExtrapMethod=Clip  InternalRulePriority=Speed  RndMeth=Simplest  InputSameDT=on
  vRef1 : InportShadow  Port=3
  vRef2 : InportShadow  Port=3
  OTL_Valid : Outport
  OTL_C3 : Outport  Port=2
  OTL_C2 : Outport  Port=3
  OTL_C1 : Outport  Port=4
  OTL_C0 : Outport  Port=5
  OTL_Range : Outport  Port=6
  TJA_Line_State : Outport  Port=7
  Line_source : Outport  Port=8
  wires:
  [SpeedKph] -> preDisMinTable7/1, preDisMinTable5/1
  preDisMinTable7/1 -> LineSelect1/27(SingleLine_DOPOut_C1)
  preDisMinTable5/1 -> LineSelect1/28(DoubleLine_DOPOut_C1)
  preDisMinTable2/1 -> MATLAB Function/7(DOP_C2_EN_Limit)
  preDisMinTable1/1 -> MATLAB Function/6(DOP_C1_EN_Limit)
  preDisMinTable3/1 -> MATLAB Function/9(DOP_C1_out_Limit)
  [SpeedKph] -> preDisMinTable1/1, preDisMinTable2/1, preDisMinTable3/1, preDisMinTable4/1
  Unit Delay2/1 -> MATLAB Function/14(dy_pre)
  LineSelect1/7(dy_pre) -> Unit Delay2/1
  Unit Delay1/1 -> MATLAB Function/15(Y_DOP)
  LineSelect1/5(Cent2DOP_flag) -> TJA_Line_Select/6(Cent2DOP_flag)
  LineSelect1/6(DOP2Cent_flag) -> TJA_Line_Select/2(DOP2Cent_flag)
  Unit Delay/1 -> MATLAB Function/1(TJA_Line)
  MATLAB Function/2(DOP_Out_Enable) -> LineSelect1/31(DOP_OUT)  "LSM_DOP_Out"
  Constant23/1 -> Relational Operator3/2
  Constant22/1 -> MATLAB Function/12(DOP_Out_Pre2Dop_Dis)
  Constant21/1 -> LineSelect1/26(SingleLine_Dop2Cent_Dislimit)
  Constant18/1 -> LineSelect1/25(SingleLine_Curr2Cent_Dislimit)
  Constant17/1 -> LineSelect1/24(SingleLine_Pre2Cent_Dislimit)
  Constant16/1 -> LineSelect1/23(SingleLine_Cent2Edge_Dislimit)
  Subtract/1 -> Line_source/1
  Constant15/1 -> Subtract/1
  LineSelect1/4(DOP2Off_flag) -> TJA_Line_Select/3(DOP2Off_flag)
  LineSelect1/3(Cent2Off_flag) -> TJA_Line_Select/1(Cent2Off_flag)
  LineSelect1/2(Off2DOP_flag) -> TJA_Line_Select/5(Off2DOP_flag)
  LineSelect1/1(Off2Cent_flag) -> TJA_Line_Select/4(Off2Cent_flag)
  kap/1 -> LineSelect1/3(kap)
  Constant13/1 -> LineSelect1/22(DoubleLine_Dop2Cent_Dislimit)
  Constant20/1 -> LineSelect1/21(DoubleLine_Curr2Cent_Dislimit)
  Constant19/1 -> LineSelect1/20(DoubleLine_Pre2Cent_Dislimit)
  EdgeLine/1 -> Bus Selector1/1
  Bus Selector1/1 -> LineSelect1/15(VisEdgeConf)  "<EdgeConf>"
  Bus Selector1/3 -> LineSelect1/17(VisEdgeA2)  "<EdgeA2>"
  Bus Selector1/5 -> LineSelect1/19(VisEdgeA0)  "<EdgeA0>"
  Bus Selector1/2 -> LineSelect1/16(VisEdgeA3)  "<EdgeA3>"
  Bus Selector1/4 -> LineSelect1/18(VisEdgeA1)  "<EdgeA1>"
  [DOP_C2] -> LineSelect1/12(bOTL)
  [DOP_C1] -> LineSelect1/13(cOTL)
  [DOP_C0] -> LineSelect1/14(dOTL)
  [DOP_C3] -> LineSelect1/11(aOTL)
  Bus Selector6/3 -> LineSelect1/7(CentLineA2)  "<CentLineC2>"
  Bus Selector6/6 -> LineSelect1/10(CentRange)  "<CentLineRange>"
  Bus Selector6/5 -> LineSelect1/9(CentLineA0)  "<CentLineC0>"
  Bus Selector6/1 -> LineSelect1/5(CentLaneValid)  "<CentLineConf>"
  Bus Selector6/2 -> LineSelect1/6(CentLineA3)  "<CentLineC3>"
  Bus Selector6/4 -> LineSelect1/8(CentLineA1)  "<CentLineC1>"
  CentLine/1 -> Bus Selector6/1
  Constant14/1 -> MATLAB Function/11(DOP_In_Pre2Dop_Dis)
  LineSelect1/8(Y_DOP) -> Unit Delay1/1
  DOP_Valid2/1 -> Compare To Constant1/1
  Line_State/1 -> LineSelect1/2(Line_State)
  Gain1/1 -> Gain2/1
  Sum1/1 -> preDisMinTable/1
  vRef2/1 -> Gain1/1
  Gain2/1 -> Sum1/1
  Constant11/1 -> Sum1/2
  LCKSts/1 -> LineSelect1/4(LCKSts)
  preDisMinTable/1 -> LineSelect1/1(Pre_dis)
  Constant9/1 -> Sum/2
  vRef1/1 -> Gain3/1
  Gain4/1 -> Sum/1
  Gain3/1 -> Gain4/1
  Sum/1 -> [SpeedKph], LineSelect1/29(Vehicle_Speed)
  Relational Operator3/1 -> MATLAB Function/13(DOP_Valid)
  MATLAB Function/1(DOP_In_Enable) -> Switch/3
  TrueDurationTime8/1 -> Relational Operator3/1
  DOP_Valid1/1 -> TrueDurationTime8/1
  preDisMinTable4/1 -> MATLAB Function/10(DOP_C2_out_Limit)
  Constant6/1 -> MATLAB Function/8(DOP_CO_out_Limit)
  Constant3/1 -> MATLAB Function/5(DOP_CO_EN_Limit)
  TJA_Line_Select/1(TJA_Line) -> Unit Delay/1, TJA_Line_State/1, Subtract/2
  DOP_C6/1 -> MATLAB Function/4(DOP_C2)
  DOP_C5/1 -> MATLAB Function/3(DOP_C1)
  DOP_C4/1 -> MATLAB Function/2(DOP_CO)
  Constant/1 -> Compare To Constant/1
  Compare To Constant/1 -> Switch/2
  Constant1/1 -> Switch/1
  Switch/1 -> LineSelect1/30(DOP_EN)  "LSM_DOP_EN"
  Logical Operator/1 -> Terminator/1
  DOP_C0/1 -> Subsystem3/1("Input "), OTL_C0/1, [DOP_C0]
  DOP_Valid/1 -> OTL_Valid/1
  Compare To Constant1/1 -> Logical Operator/1
  vRef/1 -> Gain/1
  Constant2/1 -> Max/2
  Gain/1 -> Max/1
  DOP_Range/1 -> OTL_Range/1, Relational Operator/1, [DOP_Range]
  Max/1 -> Relational Operator/2
  Relational Operator/1 -> [DOP_RangeEnable]
  [DOP_RangeEnable] -> TrueDurationTime1/1
  [DOP_C0] -> Abs/1
  Relational Operator1/1 -> Logical Operator/3  "LSM_DOP_C0MaxEnable"
  C0max/1 -> Relational Operator1/2
  Relational Operator2/1 -> Logical Operator/4  "LSM_DOP_C1MaxEnable"
  [DOP_C1] -> Abs1/1
  C1max:30°/1 -> Relational Operator2/2
  Chart/1(DopEnable) -> Logical Operator/5
  C0th/1 -> Relational Operator4/2
  [DOP_C0] -> Abs3/1
  Relational Operator4/1 -> TrueDurationTime2/1
  C1th:10°/1 -> Relational Operator5/2
  [DOP_C1] -> Abs4/1
  Relational Operator5/1 -> TrueDurationTime4/1
  Relational Operator6/1 -> TrueDurationTime6/1
  [DOP_C2] -> Abs5/1
  C2th/1 -> Relational Operator6/2
  DOP_C1/1 -> OTL_C1/1, [DOP_C1], Subsystem1/1("Input ")
  Subsystem1/1(dInput) -> [dC1]
  Subsystem2/1(dInput) -> [dC2]
  DOP_C2/1 -> OTL_C2/1, [DOP_C2], Subsystem2/1("Input ")
  Abs/1 -> Relational Operator1/1
  Abs1/1 -> Relational Operator2/1
  Abs3/1 -> Relational Operator4/1
  Abs4/1 -> Relational Operator5/1
  Abs5/1 -> Relational Operator6/1
  [dC0] -> Abs6/1
  dC0th/1 -> Relational Operator7/2
  Abs6/1 -> Relational Operator7/1
  [dC1] -> Abs7/1
  Abs7/1 -> Relational Operator8/1
  dC1th:2.5°/s/1 -> Relational Operator8/2
  [dC2] -> Abs8/1
  Abs8/1 -> Relational Operator9/1
  dC2th/1 -> Relational Operator9/2
  TrueDurationTime2/1 -> Compare To Constant2/1
  Relational Operator7/1 -> TrueDurationTime3/1
  TrueDurationTime4/1 -> Compare To Constant4/1
  Relational Operator8/1 -> TrueDurationTime5/1
  TrueDurationTime6/1 -> Compare To Constant6/1
  Relational Operator9/1 -> TrueDurationTime7/1
  Compare To Constant2/1 -> Logical Operator2/1  "LSM_DOP_C0Disable"
  Compare To Constant3/1 -> Logical Operator2/2  "LSM_DOP_dC0Disable"
  Compare To Constant4/1 -> Logical Operator2/3  "LSM_DOP_C1Disable"
  Compare To Constant5/1 -> Logical Operator2/4  "LSM_DOP_dC1Disable"
  Compare To Constant6/1 -> Logical Operator2/5  "LSM_DOP_C2Disable"
  Compare To Constant7/1 -> Logical Operator2/6  "LSM_DOP_dC2Disable"
  Subsystem3/1(dInput) -> [dC0]
  TrueDurationTime1/1 -> Compare To Constant8/1
  Compare To Constant8/1 -> Logical Operator/2  "LSM_DOP_RangeEnable"
  DOP_C3/1 -> OTL_C3/1, [DOP_C3]
  TrueDurationTime3/1 -> Compare To Constant3/1
  TrueDurationTime5/1 -> Compare To Constant5/1
  TrueDurationTime7/1 -> Compare To Constant7/1
  Relational Operator15/1 -> Compare To Constant14/1
  Relational Operator14/1 -> Compare To Constant12/1
  Relational Operator13/1 -> Compare To Constant10/1
  Compare To Constant14/1 -> Logical Operator3/6  "LSM_DOP_dC2Enable"
  Compare To Constant13/1 -> Logical Operator3/5  "LSM_DOP_C2Enable"
  Compare To Constant12/1 -> Logical Operator3/4  "LSM_DOP_dC1Enable"
  Compare To Constant11/1 -> Logical Operator3/3  "LSM_DOP_C1Enable"
  Compare To Constant10/1 -> Logical Operator3/2  "LSM_DOP_dC0Enable"
  Compare To Constant9/1 -> Logical Operator3/1  "LSM_DOP_C0Enable"
  Relational Operator12/1 -> Compare To Constant13/1
  Relational Operator11/1 -> Compare To Constant11/1
  Relational Operator10/1 -> Compare To Constant9/1
  dC2th1/1 -> Relational Operator15/2
  Abs14/1 -> Relational Operator15/1
  [dC2] -> Abs14/1
  dC1th:2.5°/s1/1 -> Relational Operator14/2
  Abs13/1 -> Relational Operator14/1
  [dC1] -> Abs13/1
  Abs12/1 -> Relational Operator13/1
  dC0th1/1 -> Relational Operator13/2
  [dC0] -> Abs12/1
  Abs11/1 -> Relational Operator12/1
  Abs10/1 -> Relational Operator11/1
  Abs9/1 -> Relational Operator10/1
  C2th1/1 -> Relational Operator12/2
  [DOP_C2] -> Abs11/1
  [DOP_C1] -> Abs10/1
  C1th:10°1/1 -> Relational Operator11/2
  [DOP_C0] -> Abs9/1
  C0th1/1 -> Relational Operator10/2
  Logical Operator2/1 -> Chart/2(Disable)
  Logical Operator3/1 -> Chart/1(Enable)
